simulink subsystem "StateSpaceControllerNominal_SubSystem"  (R2020b)
settings: Solver=VariableStepAuto  StartTime=0.0  StopTime=10.0  RelTol=1e-3
values from neighbouring files (symbols this model uses):
  K = dlqr(A,B,Q,R)    [StateSpaceControllerNominalScript.m]    (also in StateSpaceControllerRobustScript.m = Ke(2:end))
  Nu = xx(end)    [StateSpaceControllerNominalScript.m]    (also in StateSpaceControllerRobustScript.m)
  Nx = xx(1:end-1)    [StateSpaceControllerNominalScript.m]    (also in StateSpaceControllerRobustScript.m)
undefined symbols (not defined in the file or in its folder): drv
settings Model: Creator=umberto  LastModifiedBy=umberto

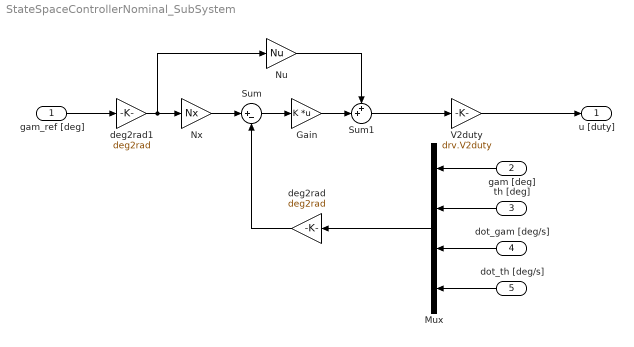
== system StateSpaceControllerNominal_SubSystem ==
  gam_ref [deg] : Inport
  gam [deg] : Inport  Port=2
  th [deg] : Inport  Port=3
  dot_gam [deg/s] : Inport  Port=4
  dot_th [deg/s] : Inport  Port=5
  Gain : Gain  Gain=K  Multiplication=Matrix(K*u)
  Mux : Mux
  Nu : Gain  Gain=Nu
  Nx : Gain  Gain=Nx
  Sum : Sum  Inputs=|+-
  Sum1 : Sum  Inputs=++|
  V2duty : Gain  Gain=drv.V2duty
  deg2rad : Gain  Gain=deg2rad
  deg2rad1 : Gain  Gain=deg2rad
  u [duty] : Outport
  wires:
  gam [deg]/1 -> Mux/1
  th [deg]/1 -> Mux/2
  dot_gam [deg/s]/1 -> Mux/3
  dot_th [deg/s]/1 -> Mux/4
  Mux/1 -> deg2rad/1
  gam_ref [deg]/1 -> deg2rad1/1
  V2duty/1 -> u [duty]/1
  Sum1/1 -> V2duty/1
  deg2rad/1 -> Sum/2
  Gain/1 -> Sum1/2
  Sum/1 -> Gain/1
  deg2rad1/1 -> Nu/1, Nx/1
  Nx/1 -> Sum/1
  Nu/1 -> Sum1/1
